simulink model "MotorCtrl_BLDC_Math"  (R2023b)
settings: Solver=FixedStepDiscrete  StartTime=0.0  StopTime=5  FixedStep=MC_Sim_BaseStep  RelTol=1e-3  EnableMultiTasking=on
values from neighbouring files (symbols this model uses):
  MC_ADC_BitNum = 0.0    [MotorControlDataDictionary_Math.sldd]    (also in MotorControlDataDictionary_Physic.sldd)
  MC_ADC_Offset = 0.0    [MotorControlDataDictionary_Math.sldd]    (also in MotorControlDataDictionary_Physic.sldd)
  MC_ADC_VRef = 1.0    [MotorControlDataDictionary_Math.sldd]    (also in MotorControlDataDictionary_Physic.sldd)
  MC_CSA_Gain = 1.0    [MotorControlDataDictionary_Math.sldd]    (also in MotorControlDataDictionary_Physic.sldd)
  MC_Input_Vdc = 13.5    [MotorControlDataDictionary_Math.sldd]    (also in MotorControlDataDictionary_Physic.sldd)
  MC_MOS_DeadTime = 1.0E-6    [MotorControlDataDictionary_Math.sldd]    (also in MotorControlDataDictionary_Physic.sldd)
  MC_Motor_Mechinal_Damp = 1.0E-5    [MotorControlDataDictionary_Math.sldd]    (also in MotorControlDataDictionary_Physic.sldd)
  MC_Motor_Mechinal_Fric = 0.0    [MotorControlDataDictionary_Math.sldd]    (also in MotorControlDataDictionary_Physic.sldd)
  MC_Motor_Mechinal_Inertia = 0.0103    [MotorControlDataDictionary_Math.sldd]    (also in MotorControlDataDictionary_Physic.sldd)
  MC_Motor_Phi = 0.0059190254913385806    [MotorControlDataDictionary_Math.sldd]    (also in MotorControlDataDictionary_Physic.sldd)
  MC_Motor_Rotor_Pn = 4.0    [MotorControlDataDictionary_Math.sldd]    (also in MotorControlDataDictionary_Physic.sldd)
  MC_Motor_Stator_Ld = 5.6345E-5    [MotorControlDataDictionary_Math.sldd]    (also in MotorControlDataDictionary_Physic.sldd)
  MC_Motor_Stator_Lq = 5.6345E-5    [MotorControlDataDictionary_Math.sldd]    (also in MotorControlDataDictionary_Physic.sldd)
  MC_Motor_Stator_Rs = 0.0286    [MotorControlDataDictionary_Math.sldd]    (also in MotorControlDataDictionary_Physic.sldd)
  MC_Param_SpeedCtrl_IdMax = 60.0    [MotorControlDataDictionary_Math.sldd]    (also in MotorControlDataDictionary_Physic.sldd)
  MC_Param_SpeedCtrl_IdMin = -60.0    [MotorControlDataDictionary_Math.sldd]    (also in MotorControlDataDictionary_Physic.sldd)
  MC_Param_SpeedCtrl_IqMax = 60.0    [MotorControlDataDictionary_Math.sldd]    (also in MotorControlDataDictionary_Physic.sldd)
  MC_Param_SpeedCtrl_IqMin = -60.0    [MotorControlDataDictionary_Math.sldd]    (also in MotorControlDataDictionary_Physic.sldd)
  MC_Param_SpeedPI_Ki = 0.57248683633241571    [MotorControlDataDictionary_Math.sldd]    (also in MotorControlDataDictionary_Physic.sldd)
  MC_Param_SpeedPI_Kp = 9.1114109857344836    [MotorControlDataDictionary_Math.sldd]    (also in MotorControlDataDictionary_Physic.sldd)
  MC_Sample_CurrentNoise = 1.0E-15    [MotorControlDataDictionary_Math.sldd]    (also in MotorControlDataDictionary_Physic.sldd)
  MC_Sample_Rs = 0.002    [MotorControlDataDictionary_Math.sldd]    (also in MotorControlDataDictionary_Physic.sldd)
  MC_Sample_VbusNoise = 1.0E-15    [MotorControlDataDictionary_Math.sldd]    (also in MotorControlDataDictionary_Physic.sldd)
  MC_Sim_BaseStep = 5.0E-7    [MotorControlDataDictionary_Math.sldd]    (also in MotorControlDataDictionary_Physic.sldd)
  MC_Sim_HFTStep = 5.0E-5    [MotorControlDataDictionary_Math.sldd]    (also in MotorControlDataDictionary_Physic.sldd)
  MC_Sim_MFTStep = 0.002    [MotorControlDataDictionary_Math.sldd]    (also in MotorControlDataDictionary_Physic.sldd)
libraries: simulink x6, spsVoltageMeasurementLib x2, spsDCVoltageSourceLib x1, spsGroundLib x1, spsPermanentMagnetSynchronousMachineLib x1, spsSeriesRLCBranchLib x1, spsThreePhaseVIMeasurementLib x1, spsUniversalBridgeLib x1, sps_lib x1
settings Model: DataDictionary=MotorControlDataDictionary_Math.sldd  SimulationMode=accelerator  Creator=YXuan  LastModifiedBy=YXuan
settings SolverCC: AutoInsertRateTranBlk=on
settings OptimizationCC: DefaultParameterBehavior=Inlined  DefaultUnderspecifiedDataType=single  EnhancedBackFolding=on  PassReuseOutputArgsAs=Individual arguments  ZeroExternalMemoryAtStartup=off  ZeroInternalMemoryAtStartup=off  EfficientFloat2IntCast=on  OptimizeBlockOrder=speed  DifferentSizesBufferReuse=on  OptimizationCustomize=off  EfficientTunableParamExpr=on
settings DebuggingCC: ParameterPrecisionLossMsg=none
settings ModelReferenceCC: EnableRefExpFcnMdlSchedulingChecks=on
settings SFSimCC: MATLABDynamicMemAlloc=off
settings RTWCC: Description=Embedded Coder  SystemTargetFile=ert.tlc  GenCodeOnly=on  TemplateMakefile=ert_default_tmf  Toolchain=Microsoft Visual C++ 2022 v17.0 | nmake (64-bit Windows)
settings CodeAppCC: ForceParamTrailComments=on  IgnoreCustomStorageClasses=off  IgnoreTestpoints=on  OperatorAnnotations=on  SimulinkDataObjDesc=on  SFDataObjDesc=on  InsertBlockDesc=on
settings ERTTargetCC: TargetLangStandard=C99 (ISO)  InferredTypesCompatibility=on  GenerateSampleERTMain=on  CombineSignalStateStructs=on  SupportAbsoluteTime=off  SupportNonFinite=off  SupportComplex=off  RemoveDisableFunc=on  InlinedParameterPlacement=NonHierarchical  ERTCustomFileTemplate=example_file_process.tlc

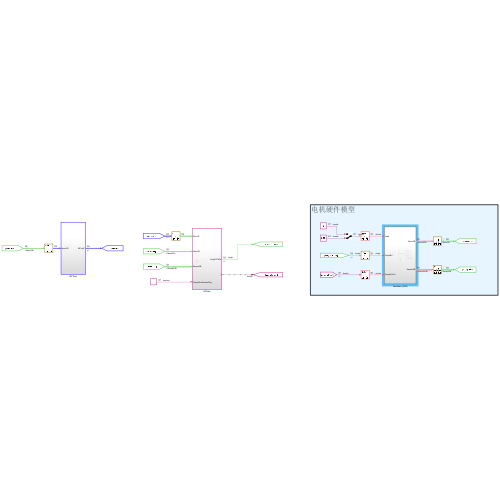
[thumbnail: Simulink's stored preview of the top-level diagram]
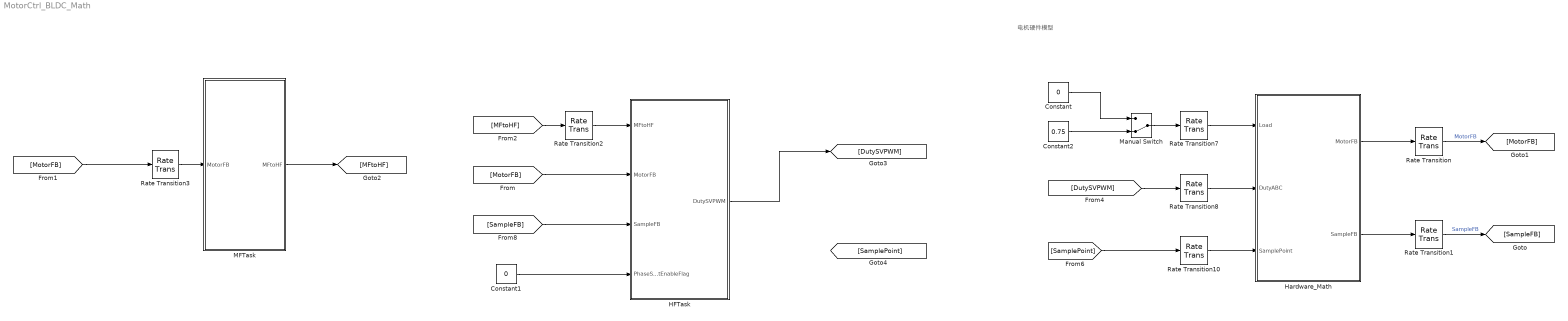
== system MotorCtrl_BLDC_Math ==
  note: 电机硬件模型
  Constant : Constant  Value=0
  Constant1 : Constant  Value=0  OutDataTypeStr=boolean
  Constant2 : Constant  Value=0.75
  HFTask : Subsystem  TreatAsAtomicUnit=on  SystemSampleTime=MC_Sim_HFTStep
  Hardware_Math : Subsystem  SystemSampleTime=MC_Sim_BaseStep  VariantControl=MC_Hardware_Motor_Model ==1&MC_Hardware_MotorMOS_Model==1
  MFTask : Subsystem  TreatAsAtomicUnit=on  SystemSampleTime=MC_Sim_MFTStep
  Manual Switch : ManualSwitch  CurrentSetting=0
  Rate Transition : RateTransition  OutPortSampleTime=MC_Sim_HFTStep
  Rate Transition1 : RateTransition  OutPortSampleTime=MC_Sim_HFTStep
  Rate Transition10 : RateTransition  OutPortSampleTime=MC_Sim_BaseStep
  Rate Transition2 : RateTransition  OutPortSampleTime=MC_Sim_HFTStep
  Rate Transition3 : RateTransition  OutPortSampleTime=MC_Sim_MFTStep
  Rate Transition7 : RateTransition  OutPortSampleTime=MC_Sim_BaseStep
  Rate Transition8 : RateTransition  OutPortSampleTime=MC_Sim_BaseStep
  wires:
  Hardware_Math/2(SampleFB) -> Rate Transition1/1
  Rate Transition8/1 -> Hardware_Math/2(DutyABC)
  Hardware_Math/1(MotorFB) -> Rate Transition/1
  [SamplePoint] -> Rate Transition10/1
  [DutySVPWM] -> Rate Transition8/1
  Rate Transition1/1 -> [SampleFB]  "SampleFB"
  Rate Transition10/1 -> Hardware_Math/3(SamplePoint)
  Rate Transition7/1 -> Hardware_Math/1(Load)
  Rate Transition/1 -> [MotorFB]  "MotorFB"
  [MotorFB] -> Rate Transition3/1
  MFTask/1(MFtoHF) -> [MFtoHF]
  [MFtoHF] -> Rate Transition2/1
  Constant1/1 -> HFTask/4(PhaseShortEnableFlag)
  [SampleFB] -> HFTask/3(SampleFB)
  [MotorFB] -> HFTask/2(MotorFB)
  HFTask/1(DutySVPWM) -> [DutySVPWM]
  ? -> [SamplePoint]
  Rate Transition2/1 -> HFTask/1(MFtoHF)
  Rate Transition3/1 -> MFTask/1(MotorFB)
  Manual Switch/1 -> Rate Transition7/1
  Constant/1 -> Manual Switch/1
  Constant2/1 -> Manual Switch/2

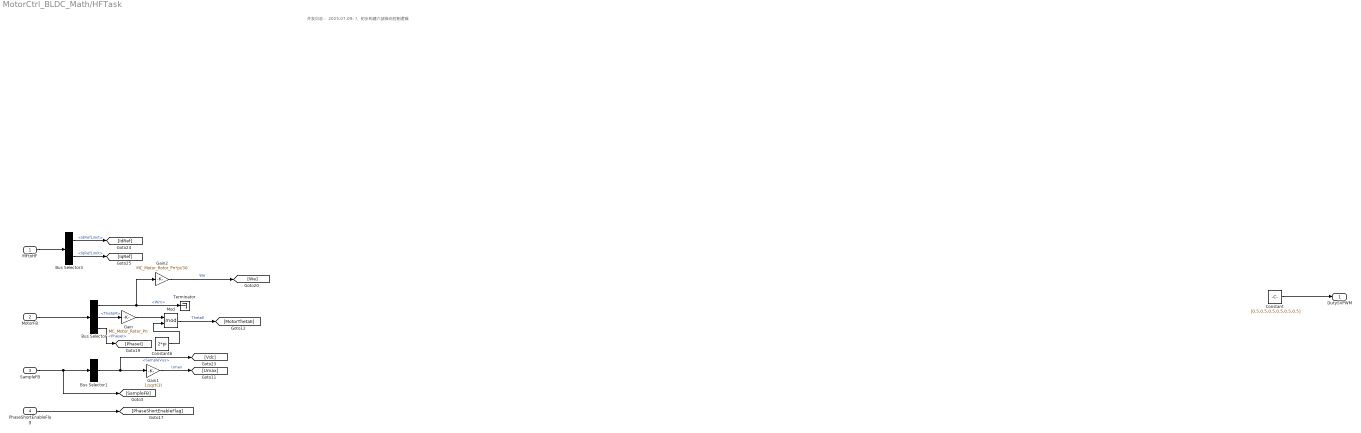
== system MotorCtrl_BLDC_Math/HFTask ==
  note: 开发日志：
      | 2025.07.09:
      | 1、初步构建六部换向控制逻辑
  MFtoHF : Inport
  MotorFB : Inport  Port=2
  SampleFB : Inport  Port=3
  PhaseShortEnableFlag : Inport  Port=4
  Bus Selector : BusSelector  OutputSignals=Wm,ThetaM,PhaseI
  Bus Selector1 : BusSelector  OutputSignals=SampleVus
  Bus Selector3 : BusSelector  OutputSignals=IdRefLimit,IqRefLimit
  Constant : Constant  Value=[0.5,0.5,0.5,0.5,0.5,0.5]  OutDataTypeStr=single
  Constant6 : Constant  Value=2*pi  OutDataTypeStr=single
  Gain : Gain  Gain=MC_Motor_Rotor_Pn  OutDataTypeStr=single
  Gain1 : Gain  Gain=1/sqrt(3)  OutDataTypeStr=single
  Gain2 : Gain  Gain=MC_Motor_Rotor_Pn*pi/30
  Mod : Math  Operator=mod
  Terminator : Terminator
  DutySVPWM : Outport
  wires:
  MFtoHF/1 -> Bus Selector3/1
  Bus Selector/2 -> Gain/1  "<ThetaM>"
  PhaseShortEnableFlag/1 -> [PhaseShortEnableFlag]
  Bus Selector/1 -> Terminator/1, Gain2/1  "<Wm>"
  Mod/1 -> [MotorThetaE]  "ThetaE"
  Bus Selector/3 -> [PhaseI]  "<PhaseI>"
  Gain/1 -> Mod/1
  Bus Selector1/1 -> [Vdc], Gain1/1  "<SampleVus>"
  SampleFB/1 -> [SampleFB], Bus Selector1/1
  Gain1/1 -> [Umax]  "Umax"
  Constant6/1 -> Mod/2
  MotorFB/1 -> Bus Selector/1
  Bus Selector3/1 -> [IdRef]  "<IdRefLimit>"
  Bus Selector3/2 -> [IqRef]  "<IqRefLimit>"
  Gain2/1 -> [We]  "We"
  Constant/1 -> DutySVPWM/1

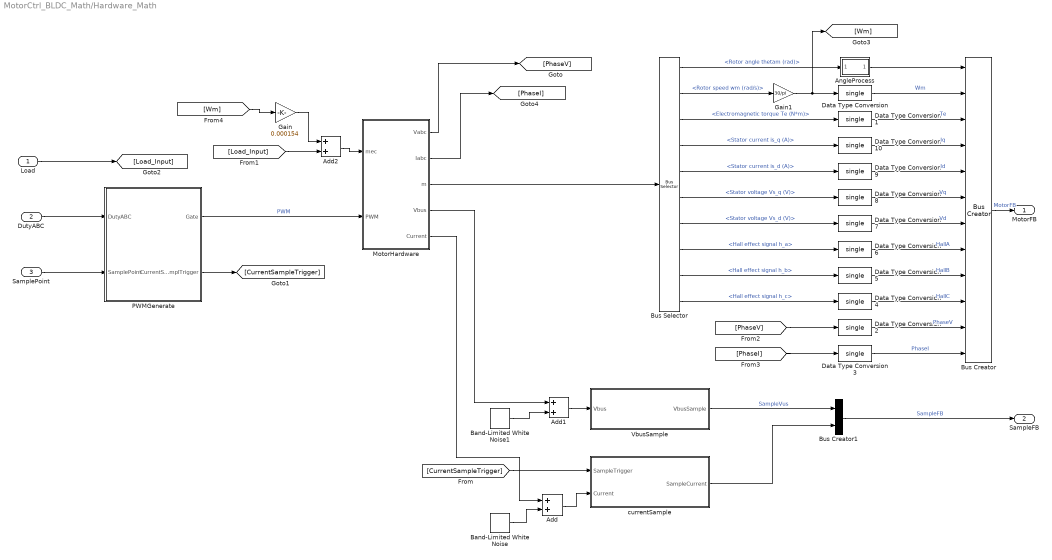
== system MotorCtrl_BLDC_Math/Hardware_Math ==
  Load : Inport
  DutyABC : Inport  Port=2
  SamplePoint : Inport  Port=3
  Add : Sum
  Add1 : Sum
  Add2 : Sum
  AngleProcess : Subsystem
  Band-Limited White Noise : simulink/Sources/Band-Limited White Noise  Cov=[MC_Sample_CurrentNoise]  Ts=MC_Sim_BaseStep  seed=[23341]
  Band-Limited White Noise1 : simulink/Sources/Band-Limited White Noise  Cov=[MC_Sample_VbusNoise]  Ts=MC_Sim_BaseStep  seed=[23341]
  Bus Creator : BusCreator  Inputs=12
  Bus Creator1 : BusCreator  Inputs=2
  Bus Selector : BusSelector  OutputSignals=Rotor angle thetam (rad),Rotor speed wm (rad/s),Electromagnetic torque Te (N*m),Stator current is_q (A),Stator current is_d (A),Stator voltage Vs_q (V),Stator voltage Vs_d (V),Hall effect signal h_a,Hall effect signal h_b,Hall effect signal h_c
  Data Type Conversion{,1..10} (11 alike) : DataTypeConversion  OutDataTypeStr=single  SaturateOnIntegerOverflow=off  RndMeth=Floor
  Gain : Gain  Gain=0.000154
  Gain1 : Gain  Gain=30/pi
  MotorHardware : Subsystem
  PWMGenerate : Subsystem  SystemSampleTime=MC_Sim_BaseStep
  VbusSample : Subsystem
  currentSample : Subsystem  Variant=on  VariantControl=Subsystem
  MotorFB : Outport
  SampleFB : Outport  Port=2
  wires:
  Band-Limited White Noise/1 -> Add/2
  Add/1 -> currentSample/2(Current)
  Add1/1 -> VbusSample/1(Vbus)
  Band-Limited White Noise1/1 -> Add1/2
  [CurrentSampleTrigger] -> currentSample/1(SampleTrigger)
  PWMGenerate/2(CurrentSamplTrigger) -> [CurrentSampleTrigger]
  Bus Selector/2 -> Gain1/1  "<Rotor speed wm (rad/s)>"
  DutyABC/1 -> PWMGenerate/1(DutyABC)
  Bus Selector/1 -> AngleProcess/1(In1)  "<Rotor angle thetam (rad)>"
  SamplePoint/1 -> PWMGenerate/2(SamplePoint)
  Bus Selector/3 -> Data Type Conversion1/1  "<Electromagnetic torque Te (N*m)>"
  Load/1 -> [Load_Input]
  Gain1/1 -> Data Type Conversion/1, [Wm]
  AngleProcess/1(Out1) -> Bus Creator/1
  [PhaseV] -> Data Type Conversion2/1
  [PhaseI] -> Data Type Conversion3/1
  VbusSample/1(VbusSample) -> Bus Creator1/1  "SampleVus"
  currentSample/1(SampleCurrent) -> Bus Creator1/2
  Bus Creator1/1 -> SampleFB/1  "SampleFB"
  PWMGenerate/1(Gate) -> MotorHardware/2(PWM)  "PWM"
  MotorHardware/1(Vabc) -> [PhaseV]
  MotorHardware/2(Iabc) -> [PhaseI]
  MotorHardware/3(m) -> Bus Selector/1
  MotorHardware/5(Current) -> Add/1
  MotorHardware/4(Vbus) -> Add1/1
  Data Type Conversion/1 -> Bus Creator/2  "Wm"
  Data Type Conversion1/1 -> Bus Creator/3  "Te"
  Data Type Conversion2/1 -> Bus Creator/11  "PhaseV"
  Data Type Conversion3/1 -> Bus Creator/12  "PhaseI"
  Bus Creator/1 -> MotorFB/1  "MotorFB"
  Add2/1 -> MotorHardware/1(mec)
  [Load_Input] -> Add2/2
  [Wm] -> Gain/1
  Gain/1 -> Add2/1
  Bus Selector/4 -> Data Type Conversion10/1  "<Stator current is_q (A)>"
  Bus Selector/5 -> Data Type Conversion9/1  "<Stator current is_d (A)>"
  Bus Selector/6 -> Data Type Conversion8/1  "<Stator voltage Vs_q (V)>"
  Bus Selector/7 -> Data Type Conversion7/1  "<Stator voltage Vs_d (V)>"
  Bus Selector/8 -> Data Type Conversion6/1  "<Hall effect signal h_a>"
  Bus Selector/9 -> Data Type Conversion5/1  "<Hall effect signal h_b>"
  Bus Selector/10 -> Data Type Conversion4/1  "<Hall effect signal h_c>"
  Data Type Conversion4/1 -> Bus Creator/10  "HallC"
  Data Type Conversion5/1 -> Bus Creator/9  "HallB"
  Data Type Conversion6/1 -> Bus Creator/8  "HallA"
  Data Type Conversion7/1 -> Bus Creator/7  "Vd"
  Data Type Conversion8/1 -> Bus Creator/6  "Vq"
  Data Type Conversion9/1 -> Bus Creator/5  "Id"
  Data Type Conversion10/1 -> Bus Creator/4  "Iq"

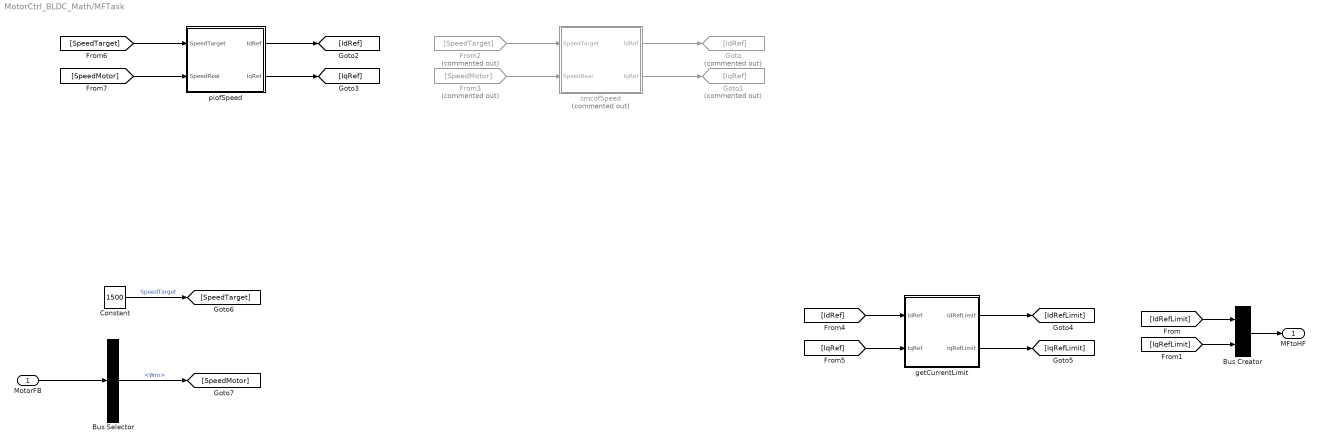
== system MotorCtrl_BLDC_Math/MFTask ==
  MotorFB : Inport
  Bus Creator : BusCreator  Inputs=2
  Bus Selector : BusSelector  OutputSignals=Wm
  Constant : Constant  Value=1500  OutDataTypeStr=single
  From2 : From  Commented=on  GotoTag=SpeedTarget
  From3 : From  Commented=on  GotoTag=SpeedMotor
  Goto : Goto  Commented=on  GotoTag=IdRef
  Goto1 : Goto  Commented=on  GotoTag=IqRef
  getCurrentLimit : Subsystem
  piofSpeed : Subsystem
  smcofSpeed : Subsystem  Commented=on
  MFtoHF : Outport
  wires:
  MotorFB/1 -> Bus Selector/1
  Bus Selector/1 -> [SpeedMotor]  "<Wm>"
  Bus Creator/1 -> MFtoHF/1
  smcofSpeed/1(IdRef) -> Goto/1
  smcofSpeed/2(IqRef) -> Goto1/1
  piofSpeed/1(IdRef) -> [IdRef]
  piofSpeed/2(IqRef) -> [IqRef]
  getCurrentLimit/2(IqRefLimit) -> [IqRefLimit]
  getCurrentLimit/1(IdRefLimit) -> [IdRefLimit]
  [IdRefLimit] -> Bus Creator/1
  [IqRefLimit] -> Bus Creator/2
  Constant/1 -> [SpeedTarget]  "SpeedTarget"
  From2/1 -> smcofSpeed/1(SpeedTarget)
  From3/1 -> smcofSpeed/2(SpeedReal)
  [IdRef] -> getCurrentLimit/1(IdRef)
  [IqRef] -> getCurrentLimit/2(IqRef)
  [SpeedTarget] -> piofSpeed/1(SpeedTarget)
  [SpeedMotor] -> piofSpeed/2(SpeedReal)

== system MotorCtrl_BLDC_Math/Hardware_Math/AngleProcess ==
  In1 : Inport
  Constant : Constant  Value=2*pi  SampleTime=-1
  Data Type Conversion : DataTypeConversion  OutDataTypeStr=single  SaturateOnIntegerOverflow=off  RndMeth=Floor
  Mod : Math  Operator=mod
  Out1 : Outport
  wires:
  Mod/1 -> Data Type Conversion/1
  In1/1 -> Mod/1
  Constant/1 -> Mod/2
  Data Type Conversion/1 -> Out1/1  "ThetaM"

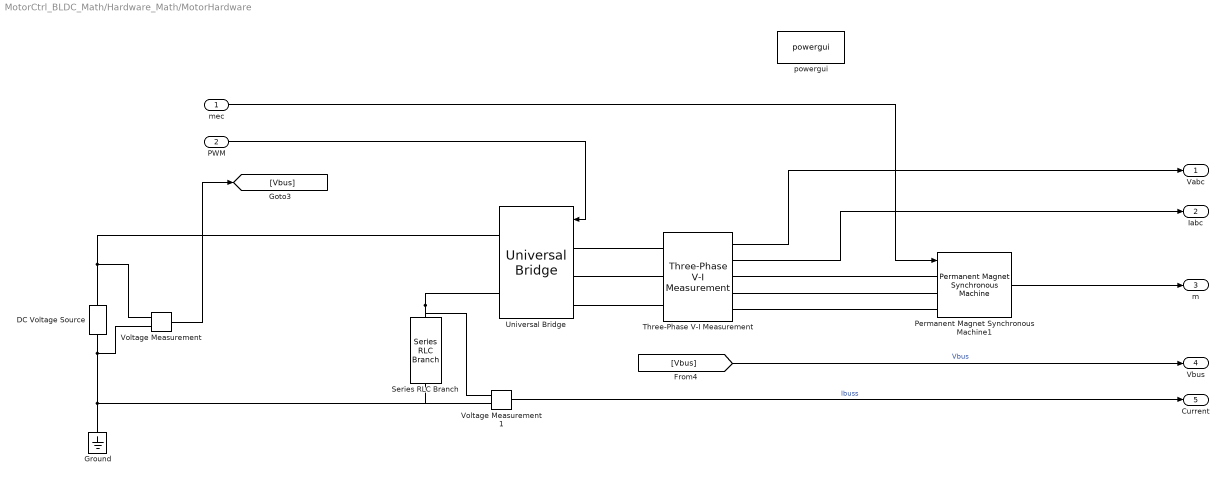
== system MotorCtrl_BLDC_Math/Hardware_Math/MotorHardware ==
  mec : Inport
  PWM : Inport  Port=2
  DC Voltage Source : spsDCVoltageSourceLib/DC Voltage Source  Amplitude=MC_Input_Vdc  Measurements=None
  Ground : spsGroundLib/Ground  LConnTagsString=a
  Permanent Magnet Synchronous Machine1 : spsPermanentMagnetSynchronousMachineLib/Permanent Magnet Synchronous Machine  NbPhases=3  FluxDistribution=Sinusoidal  RotorType=Salient-pole  MechanicalLoad=Torque Tm  PresetModel=No  ShowDetailedParameters=on  MeasurementBus=off  Resistance=MC_Motor_Stator_Rs  Inductance=8.5e-3  dqInductances=[MC_Motor_Stator_Ld MC_Motor_Stator_Lq]  La=0.000395  MachineConstant=Voltage Constant (V_peak L-L / krpm)  Flux=0.0059185  VoltageCst=MC_Motor_BEMF  TorqueCst=0.035511  Flat=120  Mechanical=[MC_Motor_Mechinal_Inertia MC_Motor_Mechinal_Damp MC_Motor_Rotor_Pn MC_Motor_Mechinal_Fric]  PolePairs=4  InitialConditions=[0,0, 0,0]  InitialConditions5ph=[0 0 0 0 0 0]  RefAngle=Aligned with phase A axis (original Park)  IterativeDiscreteModel=Trapezoidal non iterative  TsBlock=-1  TsPowergui=0
  Series RLC Branch : spsSeriesRLCBranchLib/Series RLC Branch  LConnTagsString=__new0  RConnTagsString=__new0  BranchType=R  Resistance=MC_Sample_Rs  Inductance=1e-3  SetiL0=off  InitialCurrent=0  Capacitance=1e-6  Setx0=off  InitialVoltage=0  Measurements=None
  Three-Phase V-I Measurement : spsThreePhaseVIMeasurementLib/Three-Phase V-I Measurement  VoltageMeasurement=phase-to-ground  SetLabelV=off  LabelV=Vabc  Vpu=off  VpuLL=off  CurrentMeasurement=yes  SetLabelI=off  LabelI=Iabc  Ipu=off  Pbase=100e6  Vbase=500e3  OutputType=Complex  PhasorSimulation=off  PSBequivalent=0
  Universal Bridge : spsUniversalBridgeLib/Universal Bridge  Arms=3  SnubberResistance=1e5  SnubberCapacitance=inf  Device=MOSFET / Diodes  Ron=MC_MOS_Rds  Lon=0  ForwardVoltages="[  0  0  ]"  ForwardVoltage=MC_Hardware_MOS_Threshold  GTOparameters=[ 10e-6 , 20e-6 ]  IGBTparameters=[ 1e-6 , 2e-6 ]  Measurements=None  Measurements_2=None  converterType=Rectifier
  Voltage Measurement : spsVoltageMeasurementLib/Voltage Measurement  PhasorSimulation=off  OutputType=Complex  PSBequivalent=0
  Voltage Measurement1 : spsVoltageMeasurementLib/Voltage Measurement  PhasorSimulation=off  OutputType=Complex  PSBequivalent=0
  powergui : sps_lib/powergui  Priority=1  SimulationMode=Discrete  SampleTime=MC_Sim_BaseStep  frequency=60  Iterations=50  frequencyindice=0  Pbase=100e6  ErrMax=1e-4  UnitsV=kV  UnitsW=MW  buscounter=0  FunctionMessages=off  echomessages=off  EnableUseOfTLC=off  CurrentSourceSwitches=off  DisableSnubberDevices=off  DisableRonSwitches=off  DisableVfSwitches=off  DisplayEquations=off  AutomaticDiscreteSolvers=off  SolverType=Tustin/Backward Euler (TBE)  Interpol=off  ExternalGateDelay=off  methode=off  Ts=100  x0status=blocks  SPID=on  SwTol=0  HookPort=off  NonlinearTolerance=1e-4  nMaxIteration=100  ContinueOnMaxIteration=off  RestoreLinks=warning  ResistiveCurrentMeasurement=off  Frange=[0:2:500]  Ylog=off  Xlog=on  ShowGrid=off  save=off  variable=ZData  structure=0  ZoomFFT=off  StartTime=0.0  cycles=1  DisplayStyle=1  fundamental=60  FreqAxis=off  MaxFrequency=1000  frequencyindicesteady=1  RmsSteady=1  display=off
  Vabc : Outport
  Iabc : Outport  Port=2
  m : Outport  Port=3
  Vbus : Outport  Port=4
  Current : Outport  Port=5
  wires:
  mec/1 -> Permanent Magnet Synchronous Machine1/1
  [Vbus] -> Vbus/1  "Vbus"
  Voltage Measurement/1 -> [Vbus]
  Three-Phase V-I Measurement/1 -> Vabc/1
  Three-Phase V-I Measurement/2 -> Iabc/1
  Voltage Measurement1/1 -> Current/1  "Ibuss"
  PWM/1 -> Universal Bridge/1
  Permanent Magnet Synchronous Machine1/1 -> m/1
  connections:
  Permanent Magnet Synchronous Machine1/LConn2 -- Three-Phase V-I Measurement/RConn2
  Voltage Measurement/LConn2 -- Voltage Measurement1/LConn2 -- Series RLC Branch/RConn1 -- Ground/LConn1 -- DC Voltage Source/LConn1
  Permanent Magnet Synchronous Machine1/LConn1 -- Three-Phase V-I Measurement/RConn1
  Permanent Magnet Synchronous Machine1/LConn3 -- Three-Phase V-I Measurement/RConn3
  Universal Bridge/LConn1 -- Three-Phase V-I Measurement/LConn1
  Universal Bridge/LConn2 -- Three-Phase V-I Measurement/LConn2
  Universal Bridge/LConn3 -- Three-Phase V-I Measurement/LConn3
  Voltage Measurement1/LConn1 -- Series RLC Branch/LConn1 -- Universal Bridge/RConn2
  DC Voltage Source/RConn1 -- Universal Bridge/RConn1 -- Voltage Measurement/LConn1

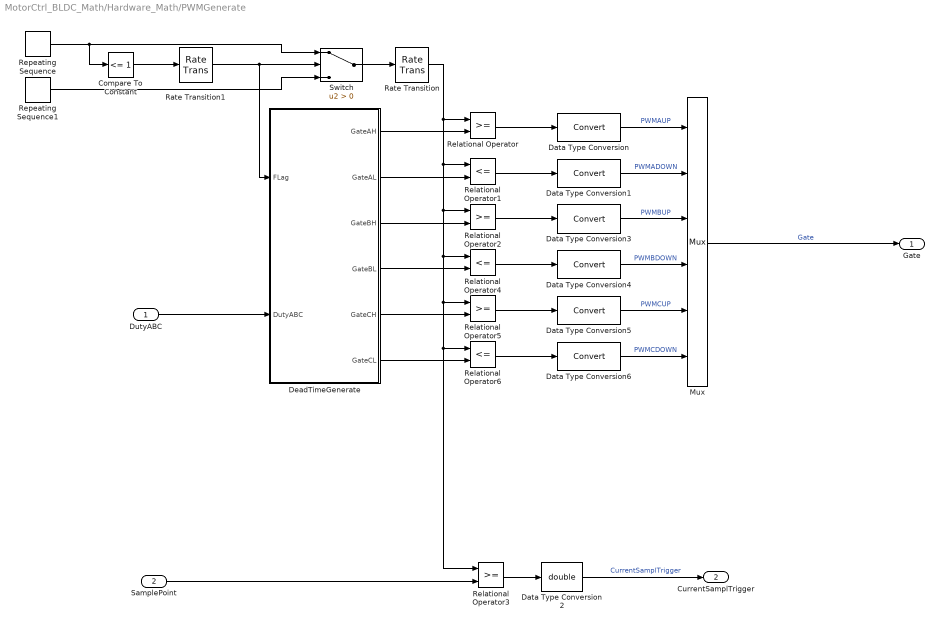
== system MotorCtrl_BLDC_Math/Hardware_Math/PWMGenerate ==
  DutyABC : Inport
  SamplePoint : Inport  Port=2
  Compare To Constant : simulink/Logic and Bit Operations/Compare To Constant  relop=<=  const=1  OutDataTypeStr=boolean
  Data Type Conversion{,1,3..6} (6 alike) : DataTypeConversion  SaturateOnIntegerOverflow=off  RndMeth=Floor
  Data Type Conversion2 : DataTypeConversion  OutDataTypeStr=double  SaturateOnIntegerOverflow=off  RndMeth=Floor
  DeadTimeGenerate : Subsystem
  Mux : Mux  Inputs=6
  Rate Transition : RateTransition  OutPortSampleTime=MC_Sim_BaseStep
  Rate Transition1 : RateTransition  OutPortSampleTime=MC_Sim_BaseStep
  Relational Operator{,2..3,5} (4 alike) : RelationalOperator  OutDataTypeStr=boolean  RndMeth=Simplest  InputSameDT=off
  Relational Operator1 : RelationalOperator  Operator=<=  OutDataTypeStr=boolean  RndMeth=Simplest  InputSameDT=off
  Relational Operator4 : RelationalOperator  Operator=<=  OutDataTypeStr=boolean  RndMeth=Simplest  InputSameDT=off
  Relational Operator6 : RelationalOperator  Operator=<=  OutDataTypeStr=boolean  RndMeth=Simplest  InputSameDT=off
  Repeating Sequence : simulink/Sources/Repeating Sequence  rep_seq_t=[0 MC_Sim_HFTStep/2 MC_Sim_HFTStep]  rep_seq_y=[0 1 2]
  Repeating Sequence1 : simulink/Sources/Repeating Sequence  rep_seq_t=[0 MC_Sim_HFTStep/2 MC_Sim_HFTStep]  rep_seq_y=[2 1 0]
  Switch : Switch  Criteria=u2 > Threshold  SaturateOnIntegerOverflow=off  InputSameDT=off
  Gate : Outport
  CurrentSamplTrigger : Outport  Port=2
  wires:
  Data Type Conversion6/1 -> Mux/6  "PWMCDOWN"
  Data Type Conversion5/1 -> Mux/5  "PWMCUP"
  Data Type Conversion4/1 -> Mux/4  "PWMBDOWN"
  Data Type Conversion3/1 -> Mux/3  "PWMBUP"
  Data Type Conversion1/1 -> Mux/2  "PWMADOWN"
  Data Type Conversion/1 -> Mux/1  "PWMAUP"
  DeadTimeGenerate/6(GateCL) -> Relational Operator6/2
  DeadTimeGenerate/5(GateCH) -> Relational Operator5/2
  DeadTimeGenerate/4(GateBL) -> Relational Operator4/2
  DeadTimeGenerate/3(GateBH) -> Relational Operator2/2
  Relational Operator6/1 -> Data Type Conversion6/1
  Relational Operator5/1 -> Data Type Conversion5/1
  Relational Operator4/1 -> Data Type Conversion4/1
  Relational Operator2/1 -> Data Type Conversion3/1
  Relational Operator1/1 -> Data Type Conversion1/1
  Relational Operator/1 -> Data Type Conversion/1
  Repeating Sequence/1 -> Switch/1, Compare To Constant/1
  Repeating Sequence1/1 -> Switch/3
  DutyABC/1 -> DeadTimeGenerate/2(DutyABC)
  DeadTimeGenerate/1(GateAH) -> Relational Operator/2
  Switch/1 -> Rate Transition/1
  DeadTimeGenerate/2(GateAL) -> Relational Operator1/2
  Relational Operator3/1 -> Data Type Conversion2/1
  SamplePoint/1 -> Relational Operator3/2
  Data Type Conversion2/1 -> CurrentSamplTrigger/1  "CurrentSamplTrigger"
  Compare To Constant/1 -> Rate Transition1/1
  Mux/1 -> Gate/1  "Gate"
  Rate Transition/1 -> Relational Operator/1, Relational Operator1/1, Relational Operator3/1, Relational Operator6/1, Relational Operator5/1, Relational Operator4/1, Relational Operator2/1
  Rate Transition1/1 -> DeadTimeGenerate/1(FLag), Switch/2

== system MotorCtrl_BLDC_Math/Hardware_Math/VbusSample ==
  Vbus : Inport
  ADCOffset : Constant  Value=0  SampleTime=-1
  ADCQuality : Gain
  Add : Sum
  Data Type Conversion3 : DataTypeConversion  OutDataTypeStr=single  SaturateOnIntegerOverflow=off  RndMeth=Floor
  VbusSample : Outport
  wires:
  Vbus/1 -> Add/2
  Add/1 -> ADCQuality/1
  ADCQuality/1 -> Data Type Conversion3/1
  ADCOffset/1 -> Add/1
  Data Type Conversion3/1 -> VbusSample/1  "PhaseI"

== system MotorCtrl_BLDC_Math/Hardware_Math/currentSample ==
  SampleTrigger : Inport
  Current : Inport  Port=2
  getCurrentSample_ORS_Double : Subsystem  VariantControl=MC_Sample_Model==1 && MC_Sample_ORSType == 2
  getCurrentSample_ORS_Single : Subsystem  VariantControl=MC_Sample_Model==1 && MC_Sample_ORSType == 1
  getCurrentSample_TRS(Three) : Subsystem  VariantControl=MC_Sample_Model==3
  getCurrentSample_TRS(Two) : Subsystem  VariantControl=MC_Sample_Model==2
  SampleCurrent : Outport

== system MotorCtrl_BLDC_Math/MFTask/getCurrentLimit ==
  IdRef : Inport
  IqRef : Inport  Port=2
  Saturation : Saturate  UpperLimit=MC_Param_SpeedCtrl_IqMax  LowerLimit=MC_Param_SpeedCtrl_IqMin
  Saturation1 : Saturate  UpperLimit=MC_Param_SpeedCtrl_IdMax  LowerLimit=MC_Param_SpeedCtrl_IdMin
  Signal Copy : SignalConversion  OverrideOpt=off
  Signal Copy1 : SignalConversion  OverrideOpt=off
  IdRefLimit : Outport
  IqRefLimit : Outport  Port=2
  wires:
  IqRef/1 -> Saturation/1
  IdRef/1 -> Saturation1/1
  Signal Copy/1 -> IdRefLimit/1  "IdRefLimit"
  Signal Copy1/1 -> IqRefLimit/1  "IqRefLimit"
  Saturation/1 -> Signal Copy1/1
  Saturation1/1 -> Signal Copy/1

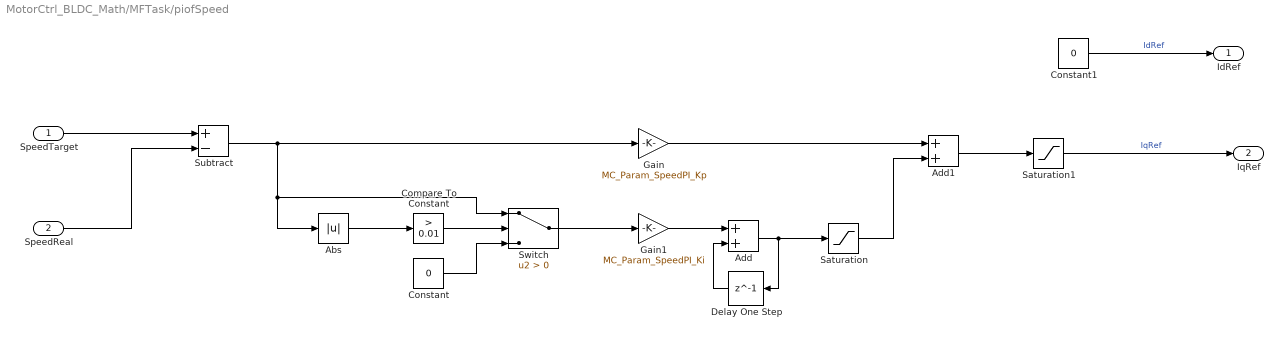
== system MotorCtrl_BLDC_Math/MFTask/piofSpeed ==
  SpeedTarget : Inport
  SpeedReal : Inport  Port=2
  Abs : Abs  SaturateOnIntegerOverflow=off
  Add : Sum
  Add1 : Sum
  Compare To Constant : simulink/Logic and Bit Operations/Compare To Constant  relop=>  const=0.01  OutDataTypeStr=boolean
  Constant : Constant  Value=0  OutDataTypeStr=single
  Constant1 : Constant  Value=0  OutDataTypeStr=single
  Delay One Step : Delay  DelayLength=1
  Gain : Gain  Gain=MC_Param_SpeedPI_Kp
  Gain1 : Gain  Gain=MC_Param_SpeedPI_Ki
  Saturation : Saturate  UpperLimit=50  LowerLimit=-50
  Saturation1 : Saturate  UpperLimit=50  LowerLimit=-50
  Subtract : Sum  Inputs=+-
  Switch : Switch  Criteria=u2 > Threshold  SaturateOnIntegerOverflow=off  InputSameDT=off
  IdRef : Outport
  IqRef : Outport  Port=2
  wires:
  Add/1 -> Saturation/1, Delay One Step/1
  Subtract/1 -> Switch/1, Abs/1, Gain/1
  Gain1/1 -> Add/1
  Saturation/1 -> Add1/2
  Delay One Step/1 -> Add/2
  Gain/1 -> Add1/1
  Compare To Constant/1 -> Switch/2
  Add1/1 -> Saturation1/1
  Abs/1 -> Compare To Constant/1
  Constant/1 -> Switch/3
  SpeedReal/1 -> Subtract/2
  SpeedTarget/1 -> Subtract/1
  Switch/1 -> Gain1/1
  Constant1/1 -> IdRef/1  "IdRef"
  Saturation1/1 -> IqRef/1  "IqRef"

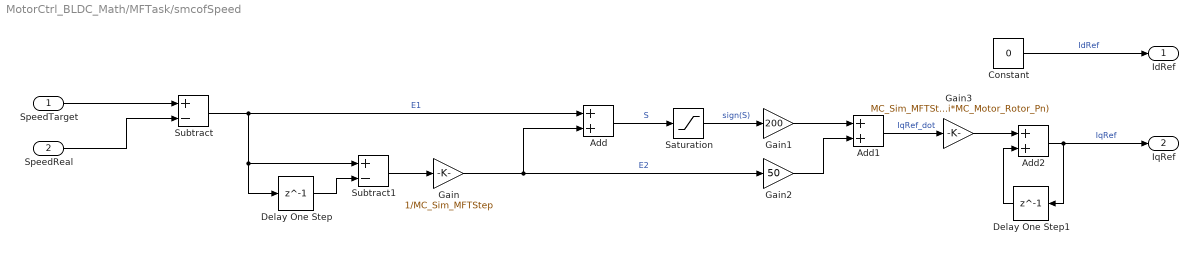
== system MotorCtrl_BLDC_Math/MFTask/smcofSpeed ==
  SpeedTarget : Inport
  SpeedReal : Inport  Port=2
  Add : Sum
  Add1 : Sum
  Add2 : Sum
  Constant : Constant  Value=0  OutDataTypeStr=single
  Delay One Step : Delay  DelayLength=1
  Delay One Step1 : Delay  DelayLength=1
  Gain : Gain  Gain=1/MC_Sim_MFTStep
  Gain1 : Gain  Gain=200
  Gain2 : Gain  Gain=50
  Gain3 : Gain  Gain=MC_Sim_MFTStep*1*MC_Motor_Mechinal_Inertia/(3*MC_Motor_Phi*MC_Motor_Rotor_Pn)
  Saturation : Saturate  UpperLimit=2  LowerLimit=-2
  Subtract : Sum  Inputs=+-
  Subtract1 : Sum  Inputs=+-
  IdRef : Outport
  IqRef : Outport  Port=2
  wires:
  SpeedTarget/1 -> Subtract/1
  SpeedReal/1 -> Subtract/2
  Subtract/1 -> Delay One Step/1, Subtract1/1, Add/1  "E1"
  Delay One Step/1 -> Subtract1/2
  Subtract1/1 -> Gain/1
  Gain/1 -> Add/2, Gain2/1  "E2"
  Add/1 -> Saturation/1  "S"
  Saturation/1 -> Gain1/1  "sign(S)"
  Gain1/1 -> Add1/1
  Gain2/1 -> Add1/2
  Add1/1 -> Gain3/1  "IqRef_dot"
  Gain3/1 -> Add2/1
  Add2/1 -> IqRef/1, Delay One Step1/1  "IqRef"
  Delay One Step1/1 -> Add2/2
  Constant/1 -> IdRef/1  "IdRef"

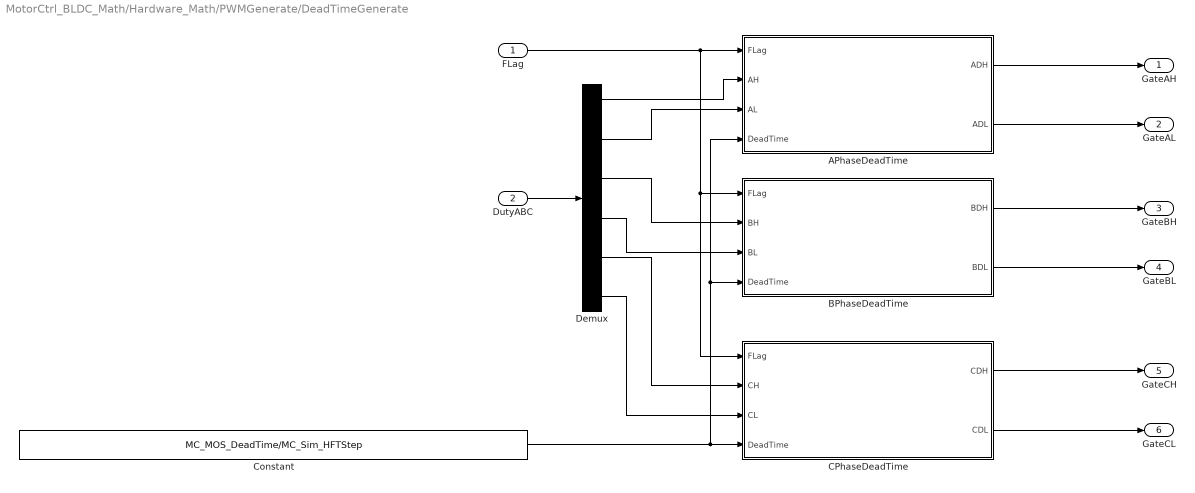
== system MotorCtrl_BLDC_Math/Hardware_Math/PWMGenerate/DeadTimeGenerate ==
  FLag : Inport
  DutyABC : Inport  Port=2
  APhaseDeadTime : Subsystem
  BPhaseDeadTime : Subsystem
  CPhaseDeadTime : Subsystem
  Constant : Constant  Value=MC_MOS_DeadTime/MC_Sim_HFTStep  SampleTime=-1
  Demux : Demux  Outputs=6
  GateAH : Outport
  GateAL : Outport  Port=2
  GateBH : Outport  Port=3
  GateBL : Outport  Port=4
  GateCH : Outport  Port=5
  GateCL : Outport  Port=6
  wires:
  Demux/6 -> CPhaseDeadTime/3(CL)
  Demux/5 -> CPhaseDeadTime/2(CH)
  Demux/4 -> BPhaseDeadTime/3(BL)
  Demux/3 -> BPhaseDeadTime/2(BH)
  Demux/2 -> APhaseDeadTime/3(AL)
  Demux/1 -> APhaseDeadTime/2(AH)
  DutyABC/1 -> Demux/1
  CPhaseDeadTime/1(CDH) -> GateCH/1
  CPhaseDeadTime/2(CDL) -> GateCL/1
  BPhaseDeadTime/1(BDH) -> GateBH/1
  BPhaseDeadTime/2(BDL) -> GateBL/1
  APhaseDeadTime/2(ADL) -> GateAL/1
  FLag/1 -> CPhaseDeadTime/1(FLag), BPhaseDeadTime/1(FLag), APhaseDeadTime/1(FLag)
  Constant/1 -> APhaseDeadTime/4(DeadTime), BPhaseDeadTime/4(DeadTime), CPhaseDeadTime/4(DeadTime)
  APhaseDeadTime/1(ADH) -> GateAH/1

== system MotorCtrl_BLDC_Math/Hardware_Math/currentSample/getCurrentSample_ORS_Double ==
  SampleTrigger : Inport
  Current : Inport  Port=2
  Demux : Demux  Outputs=2
  Mux : Mux  Inputs=2
  getCurrentSample1 : Subsystem  TreatAsAtomicUnit=on
  getCurrentSample2 : Subsystem  TreatAsAtomicUnit=on
  SampleCurrent : Outport
  wires:
  SampleTrigger/1 -> Demux/1
  Demux/1 -> getCurrentSample1/Trigger
  Demux/2 -> getCurrentSample2/Trigger
  Current/1 -> getCurrentSample2/1(Current), getCurrentSample1/1(Current)
  getCurrentSample1/1(SampleCurrentUp) -> Mux/1
  Mux/1 -> SampleCurrent/1
  getCurrentSample2/1(SampleCurrentDown) -> Mux/2

== system MotorCtrl_BLDC_Math/Hardware_Math/currentSample/getCurrentSample_ORS_Single ==
  SampleTrigger : Inport
  Current : Inport  Port=2
  Demux : Demux  Outputs=2
  Mux : Mux  Inputs=2
  getCurrentSample1 : Subsystem  TreatAsAtomicUnit=on
  getCurrentSample2 : Subsystem  TreatAsAtomicUnit=on
  SampleCurrent : Outport
  wires:
  SampleTrigger/1 -> Demux/1
  Mux/1 -> SampleCurrent/1
  getCurrentSample1/1(SampleCurrentUp) -> Mux/1
  getCurrentSample2/1(SampleCurrentDown) -> Mux/2
  Demux/1 -> getCurrentSample1/Trigger
  Demux/2 -> getCurrentSample2/Trigger
  Current/1 -> getCurrentSample2/1(Current), getCurrentSample1/1(Current)

== system MotorCtrl_BLDC_Math/Hardware_Math/currentSample/getCurrentSample_TRS(Three) ==
  SampleTrigger : Inport
  Current : Inport  Port=2
  Demux : Demux  Outputs=3
  Mux : Mux  Inputs=3
  getCurrentSampleA : Subsystem  TreatAsAtomicUnit=on
  getCurrentSampleB : Subsystem  TreatAsAtomicUnit=on
  getCurrentSampleC : Subsystem  TreatAsAtomicUnit=on
  SampleCurrent : Outport
  wires:
  getCurrentSampleA/1(SampleCurrentA) -> Mux/1
  getCurrentSampleB/1(SampleCurrentB) -> Mux/2
  Mux/1 -> SampleCurrent/1
  getCurrentSampleC/1(SampleCurrentC) -> Mux/3
  SampleTrigger/1 -> getCurrentSampleB/Trigger, getCurrentSampleC/Trigger, getCurrentSampleA/Trigger
  Current/1 -> Demux/1
  Demux/1 -> getCurrentSampleA/1(Current)
  Demux/2 -> getCurrentSampleB/1(Current)
  Demux/3 -> getCurrentSampleC/1(Current)

== system MotorCtrl_BLDC_Math/Hardware_Math/currentSample/getCurrentSample_TRS(Two) ==
  SampleTrigger : Inport
  Current : Inport  Port=2
  Demux : Demux  Outputs=2
  Mux : Mux  Inputs=2
  getCurrentSample1 : Subsystem  TreatAsAtomicUnit=on
  getCurrentSample2 : Subsystem  TreatAsAtomicUnit=on
  SampleCurrent : Outport
  wires:
  Demux/1 -> getCurrentSample1/Trigger
  Current/1 -> getCurrentSample2/1(Current), getCurrentSample1/1(Current)
  Demux/2 -> getCurrentSample2/Trigger
  getCurrentSample1/1(SampleCurrentUp) -> Mux/1
  getCurrentSample2/1(SampleCurrentDown) -> Mux/2
  Mux/1 -> SampleCurrent/1
  SampleTrigger/1 -> Demux/1

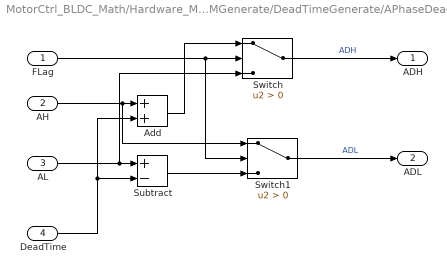
== system MotorCtrl_BLDC_Math/Hardware_Math/PWMGenerate/DeadTimeGenerate/APhaseDeadTime ==
  FLag : Inport
  AH : Inport  Port=2
  AL : Inport  Port=3
  DeadTime : Inport  Port=4
  Add : Sum
  Subtract : Sum  Inputs=+-
  Switch : Switch  Criteria=u2 > Threshold  SaturateOnIntegerOverflow=off  InputSameDT=off
  Switch1 : Switch  Criteria=u2 > Threshold  SaturateOnIntegerOverflow=off  InputSameDT=off
  ADH : Outport
  ADL : Outport  Port=2
  wires:
  DeadTime/1 -> Add/2, Subtract/2
  AL/1 -> Switch/3, Subtract/1
  FLag/1 -> Switch/2, Switch1/2
  Add/1 -> Switch/1
  Switch/1 -> ADH/1  "ADH"
  AH/1 -> Switch1/1, Add/1
  Subtract/1 -> Switch1/3
  Switch1/1 -> ADL/1  "ADL"

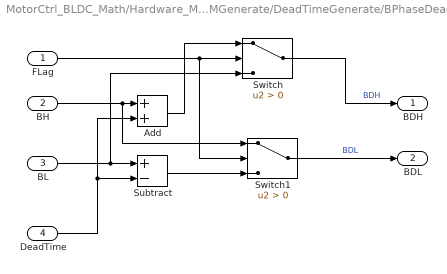
== system MotorCtrl_BLDC_Math/Hardware_Math/PWMGenerate/DeadTimeGenerate/BPhaseDeadTime ==
  FLag : Inport
  BH : Inport  Port=2
  BL : Inport  Port=3
  DeadTime : Inport  Port=4
  Add : Sum
  Subtract : Sum  Inputs=+-
  Switch : Switch  Criteria=u2 > Threshold  SaturateOnIntegerOverflow=off  InputSameDT=off
  Switch1 : Switch  Criteria=u2 > Threshold  SaturateOnIntegerOverflow=off  InputSameDT=off
  BDH : Outport
  BDL : Outport  Port=2
  wires:
  Switch1/1 -> BDL/1  "BDL"
  Subtract/1 -> Switch1/3
  BH/1 -> Switch1/1, Add/1
  Switch/1 -> BDH/1  "BDH"
  Add/1 -> Switch/1
  FLag/1 -> Switch1/2, Switch/2
  BL/1 -> Subtract/1, Switch/3
  DeadTime/1 -> Subtract/2, Add/2

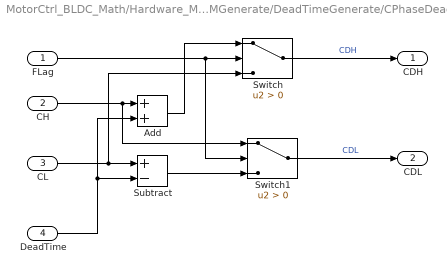
== system MotorCtrl_BLDC_Math/Hardware_Math/PWMGenerate/DeadTimeGenerate/CPhaseDeadTime ==
  FLag : Inport
  CH : Inport  Port=2
  CL : Inport  Port=3
  DeadTime : Inport  Port=4
  Add : Sum
  Subtract : Sum  Inputs=+-
  Switch : Switch  Criteria=u2 > Threshold  SaturateOnIntegerOverflow=off  InputSameDT=off
  Switch1 : Switch  Criteria=u2 > Threshold  SaturateOnIntegerOverflow=off  InputSameDT=off
  CDH : Outport
  CDL : Outport  Port=2
  wires:
  DeadTime/1 -> Add/2, Subtract/2
  CL/1 -> Switch/3, Subtract/1
  FLag/1 -> Switch/2, Switch1/2
  Add/1 -> Switch/1
  Switch/1 -> CDH/1  "CDH"
  CH/1 -> Switch1/1, Add/1
  Subtract/1 -> Switch1/3
  Switch1/1 -> CDL/1  "CDL"

== system MotorCtrl_BLDC_Math/Hardware_Math/currentSample/getCurrentSample_ORS_Double/getCurrentSample1 ==
  Current : Inport
  Trigger : TriggerPort  VariantControl=(inherit)
  ADCOffset : Constant  Value=MC_ADC_Offset  SampleTime=-1
  ADCQuality : Gain  Gain=2^MC_ADC_BitNum/MC_ADC_VRef
  Add : Sum
  CSAGain : Gain  Gain=MC_CSA_Gain
  Data Type Conversion3 : DataTypeConversion  OutDataTypeStr=single  SaturateOnIntegerOverflow=off  RndMeth=Floor
  SampleCurrentUp : Outport
  wires:
  ADCQuality/1 -> Data Type Conversion3/1
  ADCOffset/1 -> Add/1
  Add/1 -> ADCQuality/1
  CSAGain/1 -> Add/2
  Data Type Conversion3/1 -> SampleCurrentUp/1  "SampleCurrentUp"
  Current/1 -> CSAGain/1

== system MotorCtrl_BLDC_Math/Hardware_Math/currentSample/getCurrentSample_ORS_Double/getCurrentSample2 ==
  Current : Inport
  Trigger : TriggerPort  TriggerType=falling  VariantControl=(inherit)
  ADCOffset : Constant  Value=MC_ADC_Offset  SampleTime=-1
  ADCQuality : Gain  Gain=2^MC_ADC_BitNum/MC_ADC_VRef
  Add : Sum
  CSAGain : Gain  Gain=MC_CSA_Gain
  Data Type Conversion3 : DataTypeConversion  OutDataTypeStr=single  SaturateOnIntegerOverflow=off  RndMeth=Floor
  SampleCurrentDown : Outport
  wires:
  Current/1 -> CSAGain/1
  Add/1 -> ADCQuality/1
  Data Type Conversion3/1 -> SampleCurrentDown/1  "SampleCurrentUp"
  ADCOffset/1 -> Add/1
  ADCQuality/1 -> Data Type Conversion3/1
  CSAGain/1 -> Add/2

== system MotorCtrl_BLDC_Math/Hardware_Math/currentSample/getCurrentSample_ORS_Single/getCurrentSample1 ==
  Current : Inport
  Trigger : TriggerPort  VariantControl=(inherit)
  ADCOffset : Constant  Value=0  SampleTime=-1
  ADCQuality : Gain
  Add : Sum
  CSAGain : Gain
  Data Type Conversion3 : DataTypeConversion  OutDataTypeStr=single  SaturateOnIntegerOverflow=off  RndMeth=Floor
  SampleCurrentUp : Outport
  wires:
  ADCQuality/1 -> Data Type Conversion3/1
  ADCOffset/1 -> Add/1
  Add/1 -> ADCQuality/1
  CSAGain/1 -> Add/2
  Data Type Conversion3/1 -> SampleCurrentUp/1  "SampleCurrentUp"
  Current/1 -> CSAGain/1

== system MotorCtrl_BLDC_Math/Hardware_Math/currentSample/getCurrentSample_ORS_Single/getCurrentSample2 ==
  Current : Inport
  Trigger : TriggerPort  VariantControl=(inherit)
  ADCOffset : Constant  Value=0  SampleTime=-1
  ADCQuality : Gain
  Add : Sum
  CSAGain : Gain
  Data Type Conversion3 : DataTypeConversion  OutDataTypeStr=single  SaturateOnIntegerOverflow=off  RndMeth=Floor
  SampleCurrentDown : Outport
  wires:
  Current/1 -> CSAGain/1
  CSAGain/1 -> Add/2
  Add/1 -> ADCQuality/1
  ADCOffset/1 -> Add/1
  ADCQuality/1 -> Data Type Conversion3/1
  Data Type Conversion3/1 -> SampleCurrentDown/1  "SampleCurrentDown"

== system MotorCtrl_BLDC_Math/Hardware_Math/currentSample/getCurrentSample_TRS(Three)/getCurrentSampleA ==
  Current : Inport
  Trigger : TriggerPort  TriggerType=falling  VariantControl=(inherit)
  ADCOffset : Constant  Value=0  SampleTime=-1
  ADCQuality : Gain
  Add : Sum
  CSAGain : Gain
  Data Type Conversion3 : DataTypeConversion  OutDataTypeStr=single  SaturateOnIntegerOverflow=off  RndMeth=Floor
  SampleCurrentA : Outport
  wires:
  ADCQuality/1 -> Data Type Conversion3/1
  ADCOffset/1 -> Add/1
  Add/1 -> ADCQuality/1
  CSAGain/1 -> Add/2
  Data Type Conversion3/1 -> SampleCurrentA/1  "SampleCurrentA"
  Current/1 -> CSAGain/1

== system MotorCtrl_BLDC_Math/Hardware_Math/currentSample/getCurrentSample_TRS(Three)/getCurrentSampleB ==
  Current : Inport
  Trigger : TriggerPort  TriggerType=falling  VariantControl=(inherit)
  ADCOffset : Constant  Value=0  SampleTime=-1
  ADCQuality : Gain
  Add : Sum
  CSAGain : Gain
  Data Type Conversion3 : DataTypeConversion  OutDataTypeStr=single  SaturateOnIntegerOverflow=off  RndMeth=Floor
  SampleCurrentB : Outport
  wires:
  Current/1 -> CSAGain/1
  Data Type Conversion3/1 -> SampleCurrentB/1  "SampleCurrentB"
  CSAGain/1 -> Add/2
  Add/1 -> ADCQuality/1
  ADCOffset/1 -> Add/1
  ADCQuality/1 -> Data Type Conversion3/1

== system MotorCtrl_BLDC_Math/Hardware_Math/currentSample/getCurrentSample_TRS(Three)/getCurrentSampleC ==
  Current : Inport
  Trigger : TriggerPort  TriggerType=falling  VariantControl=(inherit)
  ADCOffset : Constant  Value=0  SampleTime=-1
  ADCQuality : Gain
  Add : Sum
  CSAGain : Gain
  Data Type Conversion3 : DataTypeConversion  OutDataTypeStr=single  SaturateOnIntegerOverflow=off  RndMeth=Floor
  SampleCurrentC : Outport
  wires:
  ADCQuality/1 -> Data Type Conversion3/1
  ADCOffset/1 -> Add/1
  Add/1 -> ADCQuality/1
  CSAGain/1 -> Add/2
  Data Type Conversion3/1 -> SampleCurrentC/1  "SampleCurrentC"
  Current/1 -> CSAGain/1

== system MotorCtrl_BLDC_Math/Hardware_Math/currentSample/getCurrentSample_TRS(Two)/getCurrentSample1 ==
  Current : Inport
  Trigger : TriggerPort  VariantControl=(inherit)
  ADCOffset : Constant  Value=0  SampleTime=-1
  ADCQuality : Gain
  Add : Sum
  CSAGain : Gain
  Data Type Conversion3 : DataTypeConversion  OutDataTypeStr=single  SaturateOnIntegerOverflow=off  RndMeth=Floor
  SampleCurrentUp : Outport
  wires:
  ADCQuality/1 -> Data Type Conversion3/1
  ADCOffset/1 -> Add/1
  Add/1 -> ADCQuality/1
  CSAGain/1 -> Add/2
  Data Type Conversion3/1 -> SampleCurrentUp/1  "SampleCurrentUp"
  Current/1 -> CSAGain/1

== system MotorCtrl_BLDC_Math/Hardware_Math/currentSample/getCurrentSample_TRS(Two)/getCurrentSample2 ==
  Current : Inport
  Trigger : TriggerPort  TriggerType=falling  VariantControl=(inherit)
  ADCOffset : Constant  Value=0  SampleTime=-1
  ADCQuality : Gain
  Add : Sum
  CSAGain : Gain
  Data Type Conversion3 : DataTypeConversion  OutDataTypeStr=single  SaturateOnIntegerOverflow=off  RndMeth=Floor
  SampleCurrentDown : Outport
  wires:
  Current/1 -> CSAGain/1
  Data Type Conversion3/1 -> SampleCurrentDown/1  "SampleCurrentDown"
  CSAGain/1 -> Add/2
  Add/1 -> ADCQuality/1
  ADCOffset/1 -> Add/1
  ADCQuality/1 -> Data Type Conversion3/1
